simulink model "phasor08_IEEE13"  (Simulink 10.2)
settings: Solver=ode4  StartTime=0.0  StopTime=inf  FixedStep=Ts  RelTol=1e-3  EnableMultiTasking=on
PreLoadFcn:
  | Ts=0.01;
PostLoadFcn:
  | Ts=0.01;
InitFcn:
  | Ts=0.01;
StartFcn:
  | Ts=0.01;
libraries: opal_lib x2, rtlab x2, eph_overcurrent x1, rtlab_phasor x1
settings Model: Creator=ZhiqiZhao  LastModifiedBy=xjk374
settings DataIOCC: LimitDataPoints=on
settings OptimizationCC: ExpressionDepthLimit=2147483647
settings DebuggingCC: SolverPrmCheckMsg=warning  AllowSymbolicDim=off  StateNameClashWarn=warning

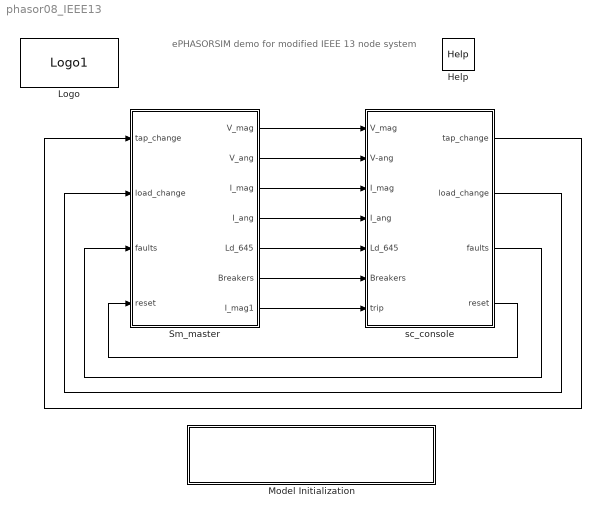
== system phasor08_IEEE13 ==
  note: ePHASORSIM demo for
      | modified IEEE 13 node system
  Help : opal_lib/Help  docfile=../help/ePH_IEEE13.html
  Logo : opal_lib/Logo1  vide=[]
  Model Initialization : Subsystem  mask(Model Functions){InitFcnX=Ts=0.01;, prel=on, posl=on, inif=on, strf=on}
      mask prompts: InitFcnX "Initialisation"; prel "Preload Function"; posl "PostLoad Function"; inif "InitFcn"; strf "StartFcn"
      mask init:
      | currentBlock = gcb;
      | root = bdroot(currentBlock);
      | 
      | if ~strcmp(get_param(root,'BlockDiagramType'),'library')
      |     if prel==1
      |         set_param(root, 'PreLoadFcn', InitFcnX);
      |     else
      |         set_param(root, 'PreLoadFcn', '');
      |     end
      |     if inif==1
      |         set_param(root, 'InitFcn', InitFcnX);
      |     else
      |         set_param(root, 'InitFcn', '');
      |     end
      |     if strf==1
      |         set_param(root, 'StartFcn', InitFcnX);
      |     else
      |         set_param(root, 'StartFcn', '');
      |     end
      |     if posl==1
      |         set_param(root, 'PostLoadFcn', InitFcnX);
      |     else
      |         set_param(root, 'PostLoadFcn', '');
      |     end
      | end
      | 
      | pos = get_param(currentBlock, 'Position');
      | width = pos(3) - pos(1); height = pos(4) - pos(2);
      | txt = [ upper(root) '\n' '- InitFcn. . . . . '  get_param(root, 'InitFcn') ];
      settings: CopyFcn=set_param(gcb,'LinkStatus','none')
      mask Display: text(5, height*0.5, txt, 'horizontalAlignment', 'left', 'verticalAlignment', 'middle') ;
  Sm_master : Subsystem
  sc_console : Subsystem
  wires:
  Sm_master/1(V_mag) -> sc_console/1(V_mag)
  Sm_master/2(V_ang) -> sc_console/2(V-ang)
  Sm_master/5(Ld_645) -> sc_console/5(Ld_645)
  sc_console/1(tap_change) -> Sm_master/1(tap_change)
  sc_console/2(load_change) -> Sm_master/2(load_change)
  Sm_master/3(I_mag) -> sc_console/3(I_mag)
  Sm_master/4(I_ang) -> sc_console/4(I_ang)
  Sm_master/6(Breakers) -> sc_console/6(Breakers)
  sc_console/3(faults) -> Sm_master/3(faults)
  Sm_master/7(I_mag1) -> sc_console/7(trip)
  sc_console/4(reset) -> Sm_master/4(reset)

== system phasor08_IEEE13/Model Initialization ==

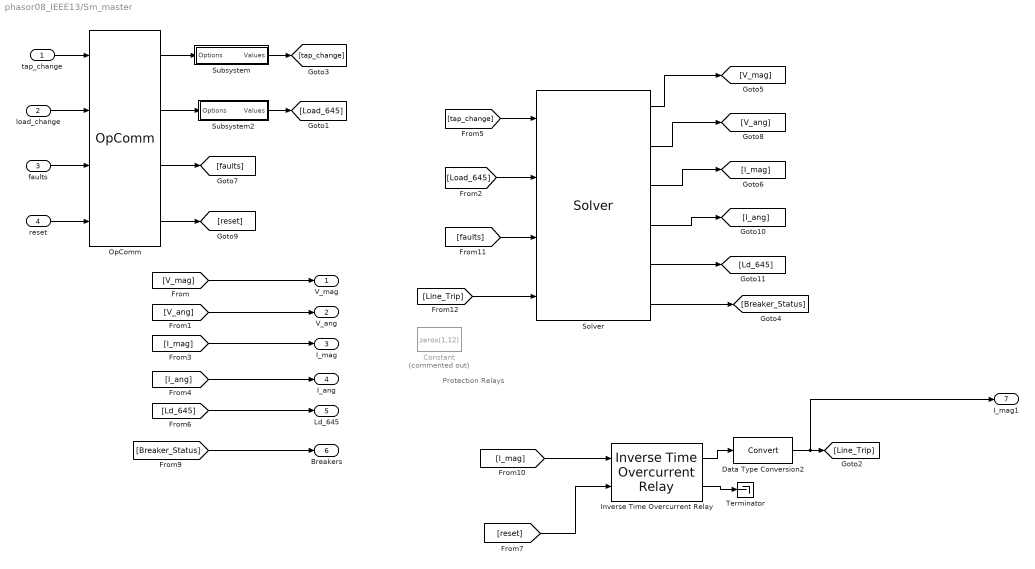
== system phasor08_IEEE13/Sm_master ==
  note: Protection
      | Relays
  tap_change : Inport
  load_change : Inport  Port=2
  faults : Inport  Port=3
  reset : Inport  Port=4
  Constant : Constant  Commented=on  Value=zeros(1,12)
  Data Type Conversion2 : DataTypeConversion
  Inverse Time Overcurrent Relay : eph_overcurrent/Inverse Time Overcurrent Relay  Ts=Ts  N=12  characteristic=6: I.E.C Class A - Standard inverse (0, 0.14, 0.02)  Ipck_51P=1000*ones(1,12)  TD51P=0.05*ones(1,12)
  OpComm : rtlab/OpComm  nbport=4  groupe_acq=1  subsys_rate=0  st=0  Synchronization=on  Interpolation=on  Threshold=1.0  Missed_Data=off  Sim_Time=off  Samples=off  dynSigOut=off  from_console=1  warning_done=off  writeOpCommFile=off  Offset=off
      settings: SourceProductName=RT-LAB
  Solver : rtlab_phasor/Solver  epname=System  extension=Excel  use_udb=off  xls='phasor08_IEEE13.xls'  raw='4992b.raw'  dyr='4992b.dyr'  fmu2builtin=off  cyme='ieee13.sxst'  cyme_pf=''  cyme_unbalanced=on  powerfactory='network.xml'  builtin=on  lazy_netlist=on  capidir='CAPI'  fmudir=''  capiprefix=capicomp_  fmuprefix=fmucomp_  logging=off  sim_mode=Dynamic simulation only (without power-flow)  dt=Ts  pf_init_method=From input data  pf_tol_v=0.000001  pf_max_it=100  pf_smart_start=off  pf_flat_start=off  pf_export=off  pfrequest=off  pf_then_dyn=off  np=1  exporty=off  optim_threads=off  perflog_on=off  script_activate_postinit=off  script_postinit_name=''
  Subsystem : Subsystem
  Subsystem2 : Subsystem
  Terminator : Terminator
  V_mag : Outport
  V_ang : Outport  Port=2
  I_mag : Outport  Port=3
  I_ang : Outport  Port=4
  Ld_645 : Outport  Port=5
  Breakers : Outport  Port=6
  I_mag1 : Outport  Port=7
  wires:
  tap_change/1 -> OpComm/1
  [tap_change] -> Solver/1
  Solver/1 -> [V_mag]
  Solver/2 -> [V_ang]
  Solver/3 -> [I_mag]
  Solver/4 -> [I_ang]
  Solver/5 -> [Ld_645]
  [Load_645] -> Solver/2
  load_change/1 -> OpComm/2
  [V_mag] -> V_mag/1
  [V_ang] -> V_ang/1
  [I_ang] -> I_ang/1
  [I_mag] -> I_mag/1
  [Ld_645] -> Ld_645/1
  OpComm/1 -> Subsystem/1(Options)
  OpComm/2 -> Subsystem2/1(Options)
  Subsystem/1(Values) -> [tap_change]
  Subsystem2/1(Values) -> [Load_645]
  Inverse Time Overcurrent Relay/2 -> Terminator/1
  [reset] -> Inverse Time Overcurrent Relay/2
  Data Type Conversion2/1 -> I_mag1/1, [Line_Trip]
  Solver/6 -> [Breaker_Status]
  [Breaker_Status] -> Breakers/1
  Inverse Time Overcurrent Relay/1 -> Data Type Conversion2/1
  [I_mag] -> Inverse Time Overcurrent Relay/1
  faults/1 -> OpComm/3
  OpComm/3 -> [faults]
  [faults] -> Solver/3
  [Line_Trip] -> Solver/4
  reset/1 -> OpComm/4
  OpComm/4 -> [reset]

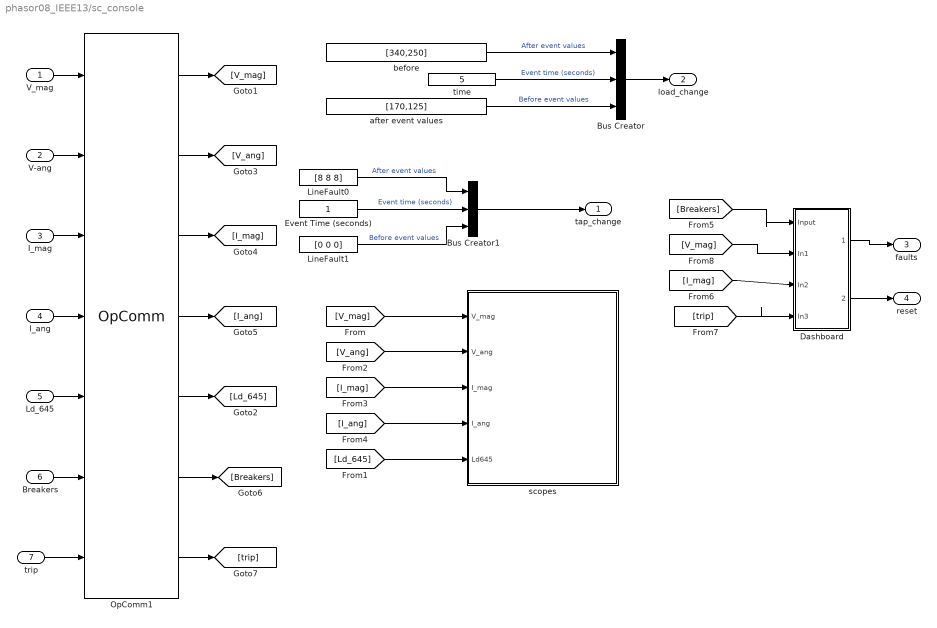
== system phasor08_IEEE13/sc_console ==
  V_mag : Inport
  V-ang : Inport  Port=2
  I_mag : Inport  Port=3
  I_ang : Inport  Port=4
  Ld_645 : Inport  Port=5
  Breakers : Inport  Port=6
  trip : Inport  Port=7
  Bus Creator : BusCreator  Inputs=3
  Bus Creator1 : BusCreator  Inputs=3
  Dashboard : Subsystem
  Event Time (seconds) : Constant
  LineFault0 : Constant  Value=[8 8 8]
  LineFault1 : Constant  Value=[0 0 0]
  OpComm1 : rtlab/OpComm  nbport=7  groupe_acq=1  subsys_rate=0  st=0  Synchronization=on  Interpolation=on  Threshold=1.0  Missed_Data=off  Sim_Time=off  Samples=off  dynSigOut=off  from_console=0  warning_done=off  writeOpCommFile=off  Offset=off
      settings: SourceProductName=RT-LAB
  after event values : Constant  Value=[170,125]
  before : Constant  Value=[340,250]
  scopes : Subsystem
  time : Constant  Value=5
  tap_change : Outport
  load_change : Outport  Port=2
  faults : Outport  Port=3
  reset : Outport  Port=4
  wires:
  V-ang/1 -> OpComm1/2
  V_mag/1 -> OpComm1/1
  OpComm1/1 -> [V_mag]
  OpComm1/2 -> [V_ang]
  time/1 -> Bus Creator/2  "Event time (seconds)"
  Bus Creator/1 -> load_change/1
  LineFault0/1 -> Bus Creator1/1  "After event values"
  LineFault1/1 -> Bus Creator1/3  "Before event values"
  Event Time (seconds)/1 -> Bus Creator1/2  "Event time (seconds)"
  Bus Creator1/1 -> tap_change/1
  before/1 -> Bus Creator/1  "After event values"
  after event values/1 -> Bus Creator/3  "Before event values"
  OpComm1/5 -> [Ld_645]
  Ld_645/1 -> OpComm1/5
  I_mag/1 -> OpComm1/3
  I_ang/1 -> OpComm1/4
  OpComm1/4 -> [I_ang]
  OpComm1/3 -> [I_mag]
  [V_mag] -> scopes/1(V_mag)
  [V_ang] -> scopes/2(V_ang)
  [I_mag] -> scopes/3(I_mag)
  [I_ang] -> scopes/4(I_ang)
  [Ld_645] -> scopes/5(Ld645)
  Breakers/1 -> OpComm1/6
  OpComm1/6 -> [Breakers]
  [Breakers] -> Dashboard/1(Input)
  Dashboard/1(Output) -> faults/1
  [I_mag] -> Dashboard/3(In2)
  trip/1 -> OpComm1/7
  OpComm1/7 -> [trip]
  [trip] -> Dashboard/4(In3)
  Dashboard/2(Output1) -> reset/1
  [V_mag] -> Dashboard/2(In1)

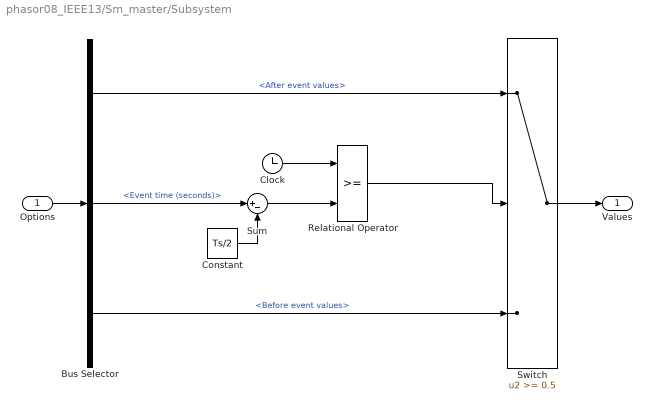
== system phasor08_IEEE13/Sm_master/Subsystem ==
  Options : Inport
  Bus Selector : BusSelector  OutputSignals=After event values,Event time (seconds),Before event values
  Clock : Clock
  Constant : Constant  Value=Ts/2
  Relational Operator : RelationalOperator  OutDataTypeStr=boolean  RndMeth=Nearest
  Sum : Sum  Inputs=|+-
  Switch : Switch  Threshold=0.5
  Values : Outport
  wires:
  Clock/1 -> Relational Operator/1
  Constant/1 -> Sum/2
  Sum/1 -> Relational Operator/2
  Bus Selector/2 -> Sum/1  "<Event time (seconds)>"
  Relational Operator/1 -> Switch/2
  Bus Selector/3 -> Switch/3  "<Before event values>"
  Bus Selector/1 -> Switch/1  "<After event values>"
  Switch/1 -> Values/1
  Options/1 -> Bus Selector/1

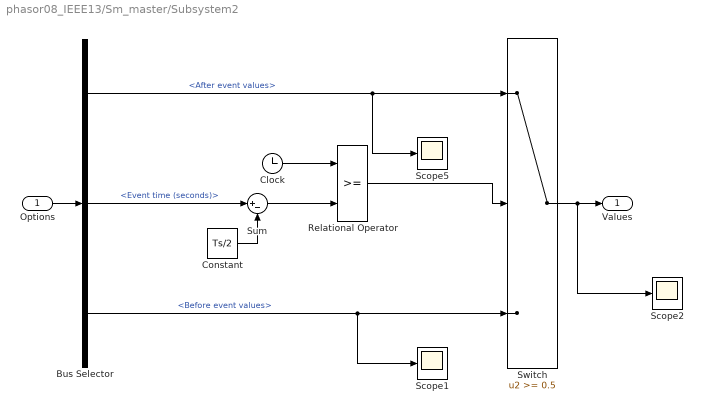
== system phasor08_IEEE13/Sm_master/Subsystem2 ==
  Options : Inport
  Bus Selector : BusSelector  OutputSignals=After event values,Event time (seconds),Before event values
  Clock : Clock
  Constant : Constant  Value=Ts/2
  Relational Operator : RelationalOperator  OutDataTypeStr=boolean  RndMeth=Nearest
  Scope1 : Scope
  Scope2 : Scope
  Scope5 : Scope
  Sum : Sum  Inputs=|+-
  Switch : Switch  Threshold=0.5
  Values : Outport
  wires:
  Clock/1 -> Relational Operator/1
  Constant/1 -> Sum/2
  Sum/1 -> Relational Operator/2
  Bus Selector/2 -> Sum/1  "<Event time (seconds)>"
  Relational Operator/1 -> Switch/2
  Bus Selector/3 -> Switch/3, Scope1/1  "<Before event values>"
  Bus Selector/1 -> Switch/1, Scope5/1  "<After event values>"
  Switch/1 -> Values/1, Scope2/1
  Options/1 -> Bus Selector/1

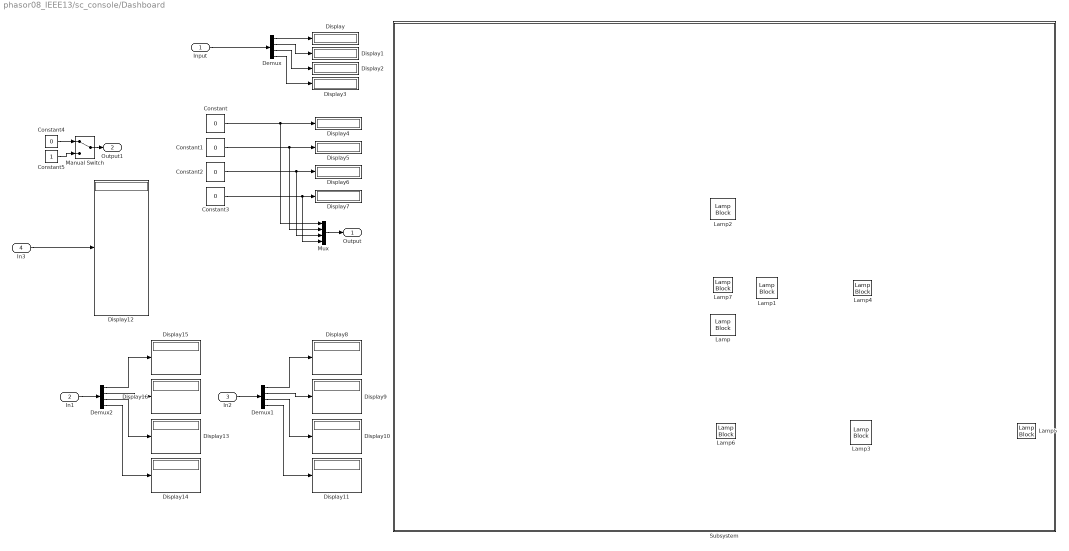
== system phasor08_IEEE13/sc_console/Dashboard ==
  Input : Inport
  In1 : Inport  Port=2
  In2 : Inport  Port=3
  In3 : Inport  Port=4
  Constant{,1..4} (5 alike) : Constant  Value=0
  Constant5 : Constant
  Demux : Demux
  Demux1 : Demux
  Demux2 : Demux
  Display{,1..16} (17 alike) : Display
  Lamp : LampBlock  LabelPosition=Hide  DefaultColor=DataTag1  States=DataTag2
  Lamp1 : LampBlock  LabelPosition=Hide  DefaultColor=DataTag4  States=DataTag5
  Lamp2 : LampBlock  LabelPosition=Hide  DefaultColor=DataTag7  States=DataTag8
  Lamp3 : LampBlock  LabelPosition=Hide  DefaultColor=DataTag10  States=DataTag11
  Lamp4 : LampBlock  LabelPosition=Hide  DefaultColor=DataTag13  States=DataTag14
  Lamp5 : LampBlock  LabelPosition=Hide  DefaultColor=DataTag16  States=DataTag17
  Lamp6 : LampBlock  LabelPosition=Hide  DefaultColor=DataTag19  States=DataTag20
  Lamp7 : LampBlock  LabelPosition=Hide  DefaultColor=DataTag22  States=DataTag23
  Manual Switch : ManualSwitch
  Mux : Mux
  Subsystem : Subsystem
      mask Display: image('C:\Users\xjk374\OneDrive\0x_Adaptive_Protection\ieee13 with relays.png'); % Use "Edit Image" on toolstrip to change.
  Output : Outport
  Output1 : Outport  Port=2
  wires:
  Demux/1 -> Display/1
  Demux/2 -> Display1/1
  Demux/3 -> Display2/1
  Demux/4 -> Display3/1
  Input/1 -> Demux/1
  Constant/1 -> Mux/1, Display4/1
  Constant1/1 -> Mux/2, Display5/1
  Constant2/1 -> Mux/3, Display6/1
  Constant3/1 -> Mux/4, Display7/1
  Mux/1 -> Output/1
  In2/1 -> Demux1/1
  Demux1/3 -> Display10/1
  Demux1/4 -> Display11/1
  Demux1/2 -> Display9/1
  Demux1/1 -> Display8/1
  In3/1 -> Display12/1
  Constant4/1 -> Manual Switch/1
  Constant5/1 -> Manual Switch/2
  Manual Switch/1 -> Output1/1
  Demux2/1 -> Display15/1
  Demux2/2 -> Display16/1
  Demux2/4 -> Display14/1
  Demux2/3 -> Display13/1
  In1/1 -> Demux2/1

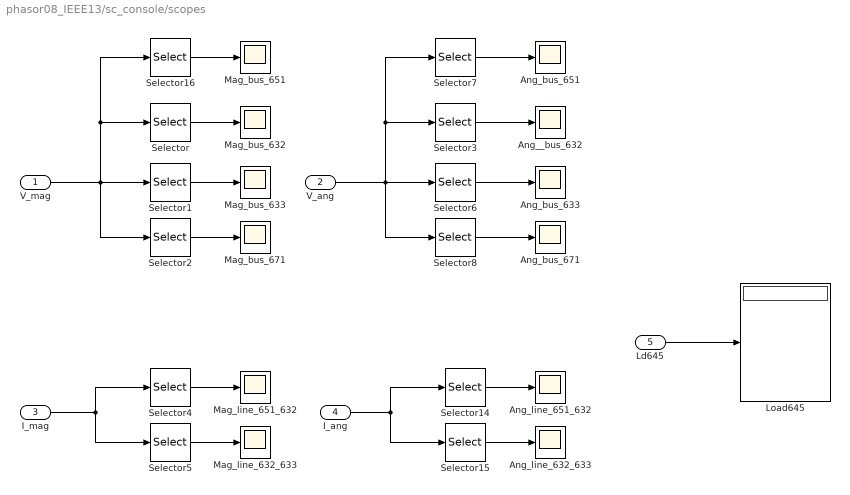
== system phasor08_IEEE13/sc_console/scopes ==
  V_mag : Inport
  V_ang : Inport  Port=2
  I_mag : Inport  Port=3
  I_ang : Inport  Port=4
  Ld645 : Inport  Port=5
  Ang__bus_632 : Scope
  Ang_bus_633 : Scope
  Ang_bus_651 : Scope
  Ang_bus_671 : Scope
  Ang_line_632_633 : Scope
  Ang_line_651_632 : Scope
  Load645 : Display
  Mag_bus_{632..633,651,671} (4 alike) : Scope
  Mag_line_632_633 : Scope
  Mag_line_651_632 : Scope
  Selector{,3,5,15} (4 alike) : Selector  InputPortWidth=12  IndexOptions=Index vector (dialog)  Indices=[4 5 6]  OutputSizes=1
  Selector1 : Selector  InputPortWidth=12  IndexOptions=Index vector (dialog)  Indices=[7 8 9]  OutputSizes=1
  Selector{4,7,14,16} (4 alike) : Selector  InputPortWidth=12  IndexOptions=Index vector (dialog)  Indices=[1 2 3]  OutputSizes=1
  Selector2 : Selector  InputPortWidth=12  IndexOptions=Index vector (dialog)  Indices=[10 11 12]  OutputSizes=1
  Selector6 : Selector  InputPortWidth=12  IndexOptions=Index vector (dialog)  Indices=[7 8 9]  OutputSizes=1
  Selector8 : Selector  InputPortWidth=12  IndexOptions=Index vector (dialog)  Indices=[10 11 12]  OutputSizes=1
  wires:
  Selector/1 -> Mag_bus_632/1
  Selector1/1 -> Mag_bus_633/1
  Selector2/1 -> Mag_bus_671/1
  V_mag/1 -> Selector1/1, Selector2/1, Selector/1, Selector16/1
  Ld645/1 -> Load645/1
  Selector4/1 -> Mag_line_651_632/1
  Selector14/1 -> Ang_line_651_632/1
  I_ang/1 -> Selector14/1, Selector15/1
  Selector16/1 -> Mag_bus_651/1
  I_mag/1 -> Selector5/1, Selector4/1
  Selector5/1 -> Mag_line_632_633/1
  Selector15/1 -> Ang_line_632_633/1
  V_ang/1 -> Selector8/1, Selector6/1, Selector7/1, Selector3/1
  Selector7/1 -> Ang_bus_651/1
  Selector3/1 -> Ang__bus_632/1
  Selector6/1 -> Ang_bus_633/1
  Selector8/1 -> Ang_bus_671/1

== system phasor08_IEEE13/sc_console/Dashboard/Subsystem ==
